simulink model "Sum17"  (Simulink 9.0)
settings: Solver=FixedStepAuto  StartTime=0.0  StopTime=10.0  FixedStep=0.1  RelTol=1e-3  EnableMultiTasking=on
settings Model: SuppressorTable=22 serialization::archive 11 0 6 0 0 0 0 0  Creator=arnaud  LastModifiedBy=hbourbou
settings DataIOCC: LimitDataPoints=on  SaveFormat=Structure  SignalLoggingSaveFormat=ModelDataLogs
settings OptimizationCC: ExpressionDepthLimit=2147483647
settings DebuggingCC: SolverPrmCheckMsg=warning  FcnCallInpInsideContextMsg=warning  StateNameClashWarn=warning
settings GRTTargetCC: GeneratePreprocessorConditionals=Disable all  CombineOutputUpdateFcns=off  GRTInterface=on
settings ConfigComp: CovSFcnEnable=off

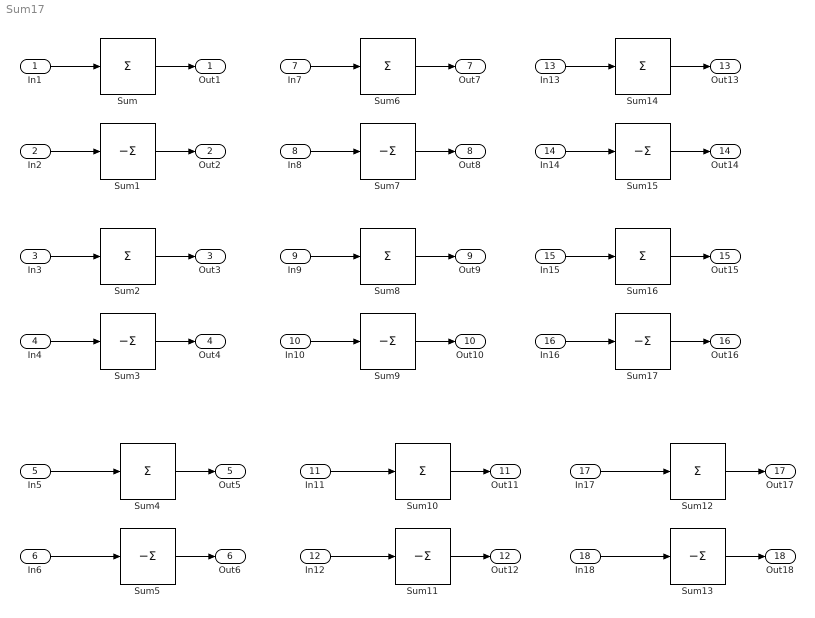
== system Sum17 ==
  In1 : Inport
  In2 : Inport  Port=2
  In3 : Inport  Port=3  PortDimensions=3
  In4 : Inport  Port=4  PortDimensions=3
  In5 : Inport  Port=5  PortDimensions=[2 3]
  In6 : Inport  Port=6  PortDimensions=[2 3]
  In7 : Inport  Port=7  OutDataTypeStr=int32
  In8 : Inport  Port=8  OutDataTypeStr=int32
  In9 : Inport  Port=9  OutDataTypeStr=int32  PortDimensions=3
  In10 : Inport  Port=10  OutDataTypeStr=int32  PortDimensions=3
  In11 : Inport  Port=11  OutDataTypeStr=int32  PortDimensions=[2 3]
  In12 : Inport  Port=12  OutDataTypeStr=int32  PortDimensions=[2 3]
  In13 : Inport  Port=13  OutDataTypeStr=int32
  In14 : Inport  Port=14  OutDataTypeStr=int32
  In15 : Inport  Port=15  OutDataTypeStr=int32  PortDimensions=3
  In16 : Inport  Port=16  OutDataTypeStr=int32  PortDimensions=3
  In17 : Inport  Port=17  OutDataTypeStr=int32  PortDimensions=[2 3]
  In18 : Inport  Port=18  OutDataTypeStr=int32  PortDimensions=[2 3]
  Sum{,2,4,6,8,10,12,14,16} (9 alike) : Sum  Inputs=+
  Sum{1,3,5,7,9,11,13,15,17} (9 alike) : Sum  Inputs=-
  Out1 : Outport
  Out2 : Outport  Port=2
  Out3 : Outport  Port=3
  Out4 : Outport  Port=4
  Out5 : Outport  Port=5
  Out6 : Outport  Port=6
  Out7 : Outport  Port=7
  Out8 : Outport  Port=8
  Out9 : Outport  Port=9
  Out10 : Outport  Port=10
  Out11 : Outport  Port=11
  Out12 : Outport  Port=12
  Out13 : Outport  Port=13
  Out14 : Outport  Port=14
  Out15 : Outport  Port=15
  Out16 : Outport  Port=16
  Out17 : Outport  Port=17
  Out18 : Outport  Port=18
  wires:
  In1/1 -> Sum/1
  Sum/1 -> Out1/1
  In7/1 -> Sum6/1
  Sum6/1 -> Out7/1
  In13/1 -> Sum14/1
  Sum14/1 -> Out13/1
  In2/1 -> Sum1/1
  Sum1/1 -> Out2/1
  In3/1 -> Sum2/1
  Sum2/1 -> Out3/1
  In4/1 -> Sum3/1
  Sum3/1 -> Out4/1
  In5/1 -> Sum4/1
  Sum4/1 -> Out5/1
  In6/1 -> Sum5/1
  Sum5/1 -> Out6/1
  In8/1 -> Sum7/1
  Sum7/1 -> Out8/1
  In9/1 -> Sum8/1
  Sum8/1 -> Out9/1
  In10/1 -> Sum9/1
  Sum9/1 -> Out10/1
  In11/1 -> Sum10/1
  Sum10/1 -> Out11/1
  In12/1 -> Sum11/1
  Sum11/1 -> Out12/1
  In14/1 -> Sum15/1
  Sum15/1 -> Out14/1
  In15/1 -> Sum16/1
  Sum16/1 -> Out15/1
  In16/1 -> Sum17/1
  Sum17/1 -> Out16/1
  In17/1 -> Sum12/1
  Sum12/1 -> Out17/1
  In18/1 -> Sum13/1
  Sum13/1 -> Out18/1
